simulink model "gm_final_heart_sym3_3_Level_fixed"  (R2021a)
settings: Solver=FixedStepDiscrete  StartTime=0.0  StopTime=8  RelTol=1e-3
libraries: hdlmdlgenlib x58
(part 2 of 3)

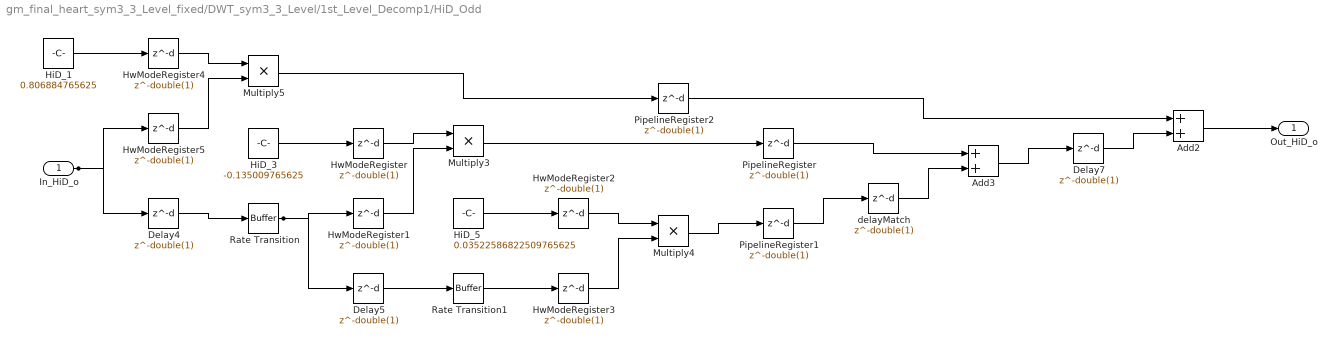
== system gm_final_heart_sym3_3_Level_fixed/DWT_sym3_3_Level/1st_Level_Decomp1/HiD_Odd ==
  In_HiD_o : Inport  OutDataTypeStr=fixdt(1, 16, 23)  PortDimensions=1  SampleTime=2.26757369614512e-05
  Add2 : Sum  AccumDataTypeStr=fixdt(1, 16, 23)  OutDataTypeStr=fixdt(1, 16, 24)  SampleTime=2.26757369614512e-05
  Add3 : Sum  AccumDataTypeStr=fixdt(1, 16, 26)  OutDataTypeStr=fixdt(1, 16, 26)  SampleTime=2.26757369614512e-05
  Delay4 : Delay  DelayLength=double(1)  InitialCondition=0  SampleTime=2.26757369614512e-05
  Delay5 : Delay  DelayLength=double(1)  InitialCondition=0  SampleTime=2.26757369614512e-05
  Delay7 : Delay  DelayLength=double(1)  InitialCondition=0  SampleTime=2.26757369614512e-05
  HiD_1 : Constant  Value=0.806884765625  OutDataTypeStr=fixdt(0, 16, 16)  SampleTime=2.26757369614512e-05
  HiD_3 : Constant  Value=-0.135009765625  OutDataTypeStr=fixdt(1, 16, 17)  SampleTime=2.26757369614512e-05
  HiD_5 : Constant  Value=0.03522586822509765625  OutDataTypeStr=fixdt(0, 16, 20)  SampleTime=2.26757369614512e-05
  HwModeRegister{,1..5} (6 alike) : Delay  DelayLength=double(1)  InitialCondition=0  SampleTime=2.26757369614512e-05
  Multiply3 : Product  Inputs=**  OutDataTypeStr=fixdt(1, 16, 15)  SampleTime=2.26757369614512e-05
  Multiply4 : Product  Inputs=**  OutDataTypeStr=fixdt(0, 16, 29)  SampleTime=2.26757369614512e-05
  Multiply5 : Product  Inputs=**  OutDataTypeStr=fixdt(0, 16, 24)  SampleTime=2.26757369614512e-05
  PipelineRegister : Delay  DelayLength=double(1)  InitialCondition=0  SampleTime=2.26757369614512e-05
  PipelineRegister1 : Delay  DelayLength=double(1)  InitialCondition=0  SampleTime=2.26757369614512e-05
  PipelineRegister2 : Delay  DelayLength=double(1)  InitialCondition=0  SampleTime=2.26757369614512e-05
  Rate Transition : hdlmdlgenlib/Buffer
      settings: SourceProductBaseCode=SL
  Rate Transition1 : hdlmdlgenlib/Buffer
      settings: SourceProductBaseCode=SL
  delayMatch : Delay  DelayLength=double(1)  InitialCondition=0  SampleTime=2.26757369614512e-05
  Out_HiD_o : Outport  OutDataTypeStr=fixdt(1,16,24)  SampleTime=2.26757369614512e-05  VectorParamsAs1DForOutWhenUnconnected=off
  wires:
  Add2/1 -> Out_HiD_o/1
  Add3/1 -> Delay7/1
  Delay4/1 -> Rate Transition/1
  Delay5/1 -> Rate Transition1/1
  Delay7/1 -> Add2/2
  HiD_1/1 -> HwModeRegister4/1
  HiD_3/1 -> HwModeRegister/1
  HiD_5/1 -> HwModeRegister2/1
  PipelineRegister/1 -> Add3/1
  delayMatch/1 -> Add3/2
  PipelineRegister2/1 -> Add2/1
  Rate Transition/1 -> Delay5/1, HwModeRegister1/1
  Rate Transition1/1 -> HwModeRegister3/1
  In_HiD_o/1 -> Delay4/1, HwModeRegister5/1
  PipelineRegister1/1 -> delayMatch/1
  Multiply3/1 -> PipelineRegister/1
  HwModeRegister/1 -> Multiply3/1
  HwModeRegister1/1 -> Multiply3/2
  Multiply4/1 -> PipelineRegister1/1
  HwModeRegister2/1 -> Multiply4/1
  HwModeRegister3/1 -> Multiply4/2
  Multiply5/1 -> PipelineRegister2/1
  HwModeRegister4/1 -> Multiply5/1
  HwModeRegister5/1 -> Multiply5/2

== system gm_final_heart_sym3_3_Level_fixed/DWT_sym3_3_Level/1st_Level_Decomp1/LoD_Even ==
  In_LoD_e : Inport  OutDataTypeStr=fixdt(1, 16, 23)  PortDimensions=1  SampleTime=2.26757369614512e-05
  Add2 : Sum  AccumDataTypeStr=fixdt(1, 16, 24)  OutDataTypeStr=fixdt(1, 16, 24)  SampleTime=2.26757369614512e-05
  Add3 : Sum  AccumDataTypeStr=fixdt(1, 16, 23)  OutDataTypeStr=fixdt(1, 16, 24)  SampleTime=2.26757369614512e-05
  Delay4 : Delay  DelayLength=double(1)  InitialCondition=0  SampleTime=2.26757369614512e-05
  Delay5 : Delay  DelayLength=double(1)  InitialCondition=0  SampleTime=2.26757369614512e-05
  Delay7 : Delay  DelayLength=double(1)  InitialCondition=0  SampleTime=2.26757369614512e-05
  HwModeRegister{,1..5} (6 alike) : Delay  DelayLength=double(1)  InitialCondition=0  SampleTime=2.26757369614512e-05
  LoD_1 : Constant  Value=0.03522586822509765625  OutDataTypeStr=fixdt(0, 16, 20)  SampleTime=2.26757369614512e-05
  LoD_3 : Constant  Value=-0.135009765625  OutDataTypeStr=fixdt(1, 16, 17)  SampleTime=2.26757369614512e-05
  LoD_5 : Constant  Value=0.806884765625  OutDataTypeStr=fixdt(0, 16, 16)  SampleTime=2.26757369614512e-05
  Multiply3 : Product  Inputs=**  OutDataTypeStr=fixdt(1, 16, 15)  SampleTime=2.26757369614512e-05
  Multiply4 : Product  Inputs=**  OutDataTypeStr=fixdt(0, 16, 24)  SampleTime=2.26757369614512e-05
  Multiply5 : Product  Inputs=**  OutDataTypeStr=fixdt(0, 16, 29)  SampleTime=2.26757369614512e-05
  PipelineRegister : Delay  DelayLength=double(1)  InitialCondition=0  SampleTime=2.26757369614512e-05
  PipelineRegister1 : Delay  DelayLength=double(1)  InitialCondition=0  SampleTime=2.26757369614512e-05
  PipelineRegister2 : Delay  DelayLength=double(1)  InitialCondition=0  SampleTime=2.26757369614512e-05
  Rate Transition : hdlmdlgenlib/Buffer
      settings: SourceProductBaseCode=SL
  Rate Transition1 : hdlmdlgenlib/Buffer
      settings: SourceProductBaseCode=SL
  delayMatch : Delay  DelayLength=double(1)  InitialCondition=0  SampleTime=2.26757369614512e-05
  Out_LoD_e : Outport  OutDataTypeStr=fixdt(1,16,24)  SampleTime=2.26757369614512e-05  VectorParamsAs1DForOutWhenUnconnected=off
  wires:
  Add2/1 -> Out_LoD_e/1
  Add3/1 -> Delay7/1
  Delay4/1 -> Rate Transition/1
  Delay5/1 -> Rate Transition1/1
  Delay7/1 -> Add2/2
  LoD_1/1 -> HwModeRegister4/1
  LoD_3/1 -> HwModeRegister/1
  LoD_5/1 -> HwModeRegister2/1
  PipelineRegister/1 -> Add3/1
  delayMatch/1 -> Add3/2
  PipelineRegister2/1 -> Add2/1
  Rate Transition/1 -> Delay5/1, HwModeRegister1/1
  Rate Transition1/1 -> HwModeRegister3/1
  In_LoD_e/1 -> Delay4/1, HwModeRegister5/1
  PipelineRegister1/1 -> delayMatch/1
  Multiply3/1 -> PipelineRegister/1
  HwModeRegister/1 -> Multiply3/1
  HwModeRegister1/1 -> Multiply3/2
  Multiply4/1 -> PipelineRegister1/1
  HwModeRegister2/1 -> Multiply4/1
  HwModeRegister3/1 -> Multiply4/2
  Multiply5/1 -> PipelineRegister2/1
  HwModeRegister4/1 -> Multiply5/1
  HwModeRegister5/1 -> Multiply5/2

== system gm_final_heart_sym3_3_Level_fixed/DWT_sym3_3_Level/1st_Level_Decomp1/LoD_Odd ==
  In_LoD_o : Inport  OutDataTypeStr=fixdt(1, 16, 23)  PortDimensions=1  SampleTime=2.26757369614512e-05
  Add2 : Sum  AccumDataTypeStr=fixdt(1, 16, 23)  OutDataTypeStr=fixdt(1, 16, 24)  SampleTime=2.26757369614512e-05
  Add3 : Sum  AccumDataTypeStr=fixdt(0, 16, 24)  OutDataTypeStr=fixdt(0, 16, 24)  SampleTime=2.26757369614512e-05
  Delay4 : Delay  DelayLength=double(1)  InitialCondition=0  SampleTime=2.26757369614512e-05
  Delay5 : Delay  DelayLength=double(1)  InitialCondition=0  SampleTime=2.26757369614512e-05
  Delay7 : Delay  DelayLength=double(1)  InitialCondition=0  SampleTime=2.26757369614512e-05
  HwModeRegister{,1..5} (6 alike) : Delay  DelayLength=double(1)  InitialCondition=0  SampleTime=2.26757369614512e-05
  LoD_1 : Constant  Value=-0.08544158935546875  OutDataTypeStr=fixdt(1, 16, 18)  SampleTime=2.26757369614512e-05
  LoD_3 : Constant  Value=0.45987701416015625  OutDataTypeStr=fixdt(0, 16, 17)  SampleTime=2.26757369614512e-05
  LoD_5 : Constant  Value=0.332672119140625  OutDataTypeStr=fixdt(0, 16, 17)  SampleTime=2.26757369614512e-05
  Multiply3 : Product  Inputs=**  OutDataTypeStr=fixdt(0, 16, 25)  SampleTime=2.26757369614512e-05
  Multiply4 : Product  Inputs=**  OutDataTypeStr=fixdt(0, 16, 26)  SampleTime=2.26757369614512e-05
  Multiply5 : Product  Inputs=**  OutDataTypeStr=fixdt(1, 16, 15)  SampleTime=2.26757369614512e-05
  PipelineRegister : Delay  DelayLength=double(1)  InitialCondition=0  SampleTime=2.26757369614512e-05
  PipelineRegister1 : Delay  DelayLength=double(1)  InitialCondition=0  SampleTime=2.26757369614512e-05
  PipelineRegister2 : Delay  DelayLength=double(1)  InitialCondition=0  SampleTime=2.26757369614512e-05
  Rate Transition : hdlmdlgenlib/Buffer
      settings: SourceProductBaseCode=SL
  Rate Transition1 : hdlmdlgenlib/Buffer
      settings: SourceProductBaseCode=SL
  delayMatch : Delay  DelayLength=double(1)  InitialCondition=0  SampleTime=2.26757369614512e-05
  Out_LoD_o : Outport  OutDataTypeStr=fixdt(1,16,24)  SampleTime=2.26757369614512e-05  VectorParamsAs1DForOutWhenUnconnected=off
  wires:
  Add2/1 -> Out_LoD_o/1
  Add3/1 -> Delay7/1
  Delay4/1 -> Rate Transition/1
  Delay5/1 -> Rate Transition1/1
  Delay7/1 -> Add2/2
  LoD_1/1 -> HwModeRegister4/1
  LoD_3/1 -> HwModeRegister/1
  LoD_5/1 -> HwModeRegister2/1
  PipelineRegister/1 -> Add3/1
  delayMatch/1 -> Add3/2
  PipelineRegister2/1 -> Add2/1
  Rate Transition/1 -> Delay5/1, HwModeRegister1/1
  Rate Transition1/1 -> HwModeRegister3/1
  In_LoD_o/1 -> Delay4/1, HwModeRegister5/1
  PipelineRegister1/1 -> delayMatch/1
  Multiply3/1 -> PipelineRegister/1
  HwModeRegister/1 -> Multiply3/1
  HwModeRegister1/1 -> Multiply3/2
  Multiply4/1 -> PipelineRegister1/1
  HwModeRegister2/1 -> Multiply4/1
  HwModeRegister3/1 -> Multiply4/2
  Multiply5/1 -> PipelineRegister2/1
  HwModeRegister4/1 -> Multiply5/1
  HwModeRegister5/1 -> Multiply5/2

== system gm_final_heart_sym3_3_Level_fixed/DWT_sym3_3_Level/1st_Level_Decomp2/HiD_Even ==
  In_HiD_e : Inport  OutDataTypeStr=fixdt(1, 16, 24)  PortDimensions=1  SampleTime=2.26757369614512e-05
  Add : Sum  AccumDataTypeStr=fixdt(1, 16, 24)  OutDataTypeStr=fixdt(1, 16, 24)  SampleTime=2.26757369614512e-05
  Add1 : Sum  AccumDataTypeStr=fixdt(1, 16, 25)  OutDataTypeStr=fixdt(1, 16, 25)  SampleTime=2.26757369614512e-05
  Delay : Delay  DelayLength=double(1)  InitialCondition=0  SampleTime=2.26757369614512e-05
  Delay1 : Delay  DelayLength=double(1)  InitialCondition=0  SampleTime=2.26757369614512e-05
  Delay3 : Delay  DelayLength=double(1)  InitialCondition=0  SampleTime=2.26757369614512e-05
  HiD_0 : Constant  Value=-0.332672119140625  OutDataTypeStr=fixdt(1, 16, 16)  SampleTime=2.26757369614512e-05
  HiD_2 : Constant  Value=-0.4598846435546875  OutDataTypeStr=fixdt(1, 16, 16)  SampleTime=2.26757369614512e-05
  HiD_4 : Constant  Value=0.08544158935546875  OutDataTypeStr=fixdt(0, 16, 19)  SampleTime=2.26757369614512e-05
  HwModeRegister{,1..5} (6 alike) : Delay  DelayLength=double(1)  InitialCondition=0  SampleTime=2.26757369614512e-05
  Multiply1 : Product  Inputs=**  OutDataTypeStr=fixdt(1, 16, 15)  SampleTime=2.26757369614512e-05
  Multiply2 : Product  Inputs=**  OutDataTypeStr=fixdt(0, 16, 28)  SampleTime=2.26757369614512e-05
  Multiply3 : Product  Inputs=**  OutDataTypeStr=fixdt(1, 16, 15)  SampleTime=2.26757369614512e-05
  PipelineRegister : Delay  DelayLength=double(1)  InitialCondition=0  SampleTime=2.26757369614512e-05
  PipelineRegister1 : Delay  DelayLength=double(1)  InitialCondition=0  SampleTime=2.26757369614512e-05
  PipelineRegister2 : Delay  DelayLength=double(1)  InitialCondition=0  SampleTime=2.26757369614512e-05
  Rate Transition : hdlmdlgenlib/Buffer
      settings: SourceProductBaseCode=SL
  Rate Transition1 : hdlmdlgenlib/Buffer
      settings: SourceProductBaseCode=SL
  delayMatch : Delay  DelayLength=double(1)  InitialCondition=0  SampleTime=2.26757369614512e-05
  Out_HiD_e : Outport  OutDataTypeStr=fixdt(1,16,24)  SampleTime=2.26757369614512e-05  VectorParamsAs1DForOutWhenUnconnected=off
  wires:
  Add/1 -> Out_HiD_e/1
  Add1/1 -> Delay3/1
  Delay/1 -> Rate Transition/1
  Delay1/1 -> Rate Transition1/1
  Delay3/1 -> Add/2
  HiD_0/1 -> HwModeRegister4/1
  HiD_2/1 -> HwModeRegister/1
  HiD_4/1 -> HwModeRegister2/1
  PipelineRegister/1 -> Add1/1
  delayMatch/1 -> Add1/2
  PipelineRegister2/1 -> Add/1
  Rate Transition/1 -> Delay1/1, HwModeRegister1/1
  Rate Transition1/1 -> HwModeRegister3/1
  In_HiD_e/1 -> Delay/1, HwModeRegister5/1
  PipelineRegister1/1 -> delayMatch/1
  Multiply1/1 -> PipelineRegister/1
  HwModeRegister/1 -> Multiply1/1
  HwModeRegister1/1 -> Multiply1/2
  Multiply2/1 -> PipelineRegister1/1
  HwModeRegister2/1 -> Multiply2/1
  HwModeRegister3/1 -> Multiply2/2
  Multiply3/1 -> PipelineRegister2/1
  HwModeRegister4/1 -> Multiply3/1
  HwModeRegister5/1 -> Multiply3/2

== system gm_final_heart_sym3_3_Level_fixed/DWT_sym3_3_Level/1st_Level_Decomp2/HiD_Odd ==
  In_HiD_o : Inport  OutDataTypeStr=fixdt(1, 16, 24)  PortDimensions=1  SampleTime=2.26757369614512e-05
  Add2 : Sum  AccumDataTypeStr=fixdt(1, 16, 24)  OutDataTypeStr=fixdt(1, 16, 24)  SampleTime=2.26757369614512e-05
  Add3 : Sum  AccumDataTypeStr=fixdt(1, 16, 26)  OutDataTypeStr=fixdt(1, 16, 27)  SampleTime=2.26757369614512e-05
  Delay4 : Delay  DelayLength=double(1)  InitialCondition=0  SampleTime=2.26757369614512e-05
  Delay5 : Delay  DelayLength=double(1)  InitialCondition=0  SampleTime=2.26757369614512e-05
  Delay7 : Delay  DelayLength=double(1)  InitialCondition=0  SampleTime=2.26757369614512e-05
  HiD_1 : Constant  Value=0.806884765625  OutDataTypeStr=fixdt(0, 16, 16)  SampleTime=2.26757369614512e-05
  HiD_3 : Constant  Value=-0.135009765625  OutDataTypeStr=fixdt(1, 16, 17)  SampleTime=2.26757369614512e-05
  HiD_5 : Constant  Value=0.03522586822509765625  OutDataTypeStr=fixdt(0, 16, 20)  SampleTime=2.26757369614512e-05
  HwModeRegister{,1..5} (6 alike) : Delay  DelayLength=double(1)  InitialCondition=0  SampleTime=2.26757369614512e-05
  Multiply3 : Product  Inputs=**  OutDataTypeStr=fixdt(1, 16, 15)  SampleTime=2.26757369614512e-05
  Multiply4 : Product  Inputs=**  OutDataTypeStr=fixdt(0, 16, 29)  SampleTime=2.26757369614512e-05
  Multiply5 : Product  Inputs=**  OutDataTypeStr=fixdt(0, 16, 25)  SampleTime=2.26757369614512e-05
  PipelineRegister : Delay  DelayLength=double(1)  InitialCondition=0  SampleTime=2.26757369614512e-05
  PipelineRegister1 : Delay  DelayLength=double(1)  InitialCondition=0  SampleTime=2.26757369614512e-05
  PipelineRegister2 : Delay  DelayLength=double(1)  InitialCondition=0  SampleTime=2.26757369614512e-05
  Rate Transition : hdlmdlgenlib/Buffer
      settings: SourceProductBaseCode=SL
  Rate Transition1 : hdlmdlgenlib/Buffer
      settings: SourceProductBaseCode=SL
  delayMatch : Delay  DelayLength=double(1)  InitialCondition=0  SampleTime=2.26757369614512e-05
  Out_HiD_o : Outport  OutDataTypeStr=fixdt(1,16,24)  SampleTime=2.26757369614512e-05  VectorParamsAs1DForOutWhenUnconnected=off
  wires:
  Add2/1 -> Out_HiD_o/1
  Add3/1 -> Delay7/1
  Delay4/1 -> Rate Transition/1
  Delay5/1 -> Rate Transition1/1
  Delay7/1 -> Add2/2
  HiD_1/1 -> HwModeRegister4/1
  HiD_3/1 -> HwModeRegister/1
  HiD_5/1 -> HwModeRegister2/1
  PipelineRegister/1 -> Add3/1
  delayMatch/1 -> Add3/2
  PipelineRegister2/1 -> Add2/1
  Rate Transition/1 -> Delay5/1, HwModeRegister1/1
  Rate Transition1/1 -> HwModeRegister3/1
  In_HiD_o/1 -> Delay4/1, HwModeRegister5/1
  PipelineRegister1/1 -> delayMatch/1
  Multiply3/1 -> PipelineRegister/1
  HwModeRegister/1 -> Multiply3/1
  HwModeRegister1/1 -> Multiply3/2
  Multiply4/1 -> PipelineRegister1/1
  HwModeRegister2/1 -> Multiply4/1
  HwModeRegister3/1 -> Multiply4/2
  Multiply5/1 -> PipelineRegister2/1
  HwModeRegister4/1 -> Multiply5/1
  HwModeRegister5/1 -> Multiply5/2

== system gm_final_heart_sym3_3_Level_fixed/DWT_sym3_3_Level/1st_Level_Decomp2/LoD_Even ==
  In_LoD_e : Inport  OutDataTypeStr=fixdt(1, 16, 24)  PortDimensions=1  SampleTime=2.26757369614512e-05
  Add2 : Sum  AccumDataTypeStr=fixdt(1, 16, 24)  OutDataTypeStr=fixdt(1, 16, 24)  SampleTime=2.26757369614512e-05
  Add3 : Sum  AccumDataTypeStr=fixdt(1, 16, 24)  OutDataTypeStr=fixdt(1, 16, 24)  SampleTime=2.26757369614512e-05
  Delay4 : Delay  DelayLength=double(1)  InitialCondition=0  SampleTime=2.26757369614512e-05
  Delay5 : Delay  DelayLength=double(1)  InitialCondition=0  SampleTime=2.26757369614512e-05
  Delay7 : Delay  DelayLength=double(1)  InitialCondition=0  SampleTime=2.26757369614512e-05
  HwModeRegister{,1..5} (6 alike) : Delay  DelayLength=double(1)  InitialCondition=0  SampleTime=2.26757369614512e-05
  LoD_1 : Constant  Value=0.03522586822509765625  OutDataTypeStr=fixdt(0, 16, 20)  SampleTime=2.26757369614512e-05
  LoD_3 : Constant  Value=-0.135009765625  OutDataTypeStr=fixdt(1, 16, 17)  SampleTime=2.26757369614512e-05
  LoD_5 : Constant  Value=0.806884765625  OutDataTypeStr=fixdt(0, 16, 16)  SampleTime=2.26757369614512e-05
  Multiply3 : Product  Inputs=**  OutDataTypeStr=fixdt(1, 16, 15)  SampleTime=2.26757369614512e-05
  Multiply4 : Product  Inputs=**  OutDataTypeStr=fixdt(0, 16, 25)  SampleTime=2.26757369614512e-05
  Multiply5 : Product  Inputs=**  OutDataTypeStr=fixdt(0, 16, 29)  SampleTime=2.26757369614512e-05
  PipelineRegister : Delay  DelayLength=double(1)  InitialCondition=0  SampleTime=2.26757369614512e-05
  PipelineRegister1 : Delay  DelayLength=double(1)  InitialCondition=0  SampleTime=2.26757369614512e-05
  PipelineRegister2 : Delay  DelayLength=double(1)  InitialCondition=0  SampleTime=2.26757369614512e-05
  Rate Transition : hdlmdlgenlib/Buffer
      settings: SourceProductBaseCode=SL
  Rate Transition1 : hdlmdlgenlib/Buffer
      settings: SourceProductBaseCode=SL
  delayMatch : Delay  DelayLength=double(1)  InitialCondition=0  SampleTime=2.26757369614512e-05
  Out_LoD_e : Outport  OutDataTypeStr=fixdt(1,16,24)  SampleTime=2.26757369614512e-05  VectorParamsAs1DForOutWhenUnconnected=off
  wires:
  Add2/1 -> Out_LoD_e/1
  Add3/1 -> Delay7/1
  Delay4/1 -> Rate Transition/1
  Delay5/1 -> Rate Transition1/1
  Delay7/1 -> Add2/2
  LoD_1/1 -> HwModeRegister4/1
  LoD_3/1 -> HwModeRegister/1
  LoD_5/1 -> HwModeRegister2/1
  PipelineRegister/1 -> Add3/1
  delayMatch/1 -> Add3/2
  PipelineRegister2/1 -> Add2/1
  Rate Transition/1 -> Delay5/1, HwModeRegister1/1
  Rate Transition1/1 -> HwModeRegister3/1
  In_LoD_e/1 -> Delay4/1, HwModeRegister5/1
  PipelineRegister1/1 -> delayMatch/1
  Multiply3/1 -> PipelineRegister/1
  HwModeRegister/1 -> Multiply3/1
  HwModeRegister1/1 -> Multiply3/2
  Multiply4/1 -> PipelineRegister1/1
  HwModeRegister2/1 -> Multiply4/1
  HwModeRegister3/1 -> Multiply4/2
  Multiply5/1 -> PipelineRegister2/1
  HwModeRegister4/1 -> Multiply5/1
  HwModeRegister5/1 -> Multiply5/2

== system gm_final_heart_sym3_3_Level_fixed/DWT_sym3_3_Level/1st_Level_Decomp2/LoD_Odd ==
  In_LoD_o : Inport  OutDataTypeStr=fixdt(1, 16, 24)  PortDimensions=1  SampleTime=2.26757369614512e-05
  Add2 : Sum  AccumDataTypeStr=fixdt(1, 16, 24)  OutDataTypeStr=fixdt(1, 16, 24)  SampleTime=2.26757369614512e-05
  Add3 : Sum  AccumDataTypeStr=fixdt(0, 16, 25)  OutDataTypeStr=fixdt(0, 16, 25)  SampleTime=2.26757369614512e-05
  Delay4 : Delay  DelayLength=double(1)  InitialCondition=0  SampleTime=2.26757369614512e-05
  Delay5 : Delay  DelayLength=double(1)  InitialCondition=0  SampleTime=2.26757369614512e-05
  Delay7 : Delay  DelayLength=double(1)  InitialCondition=0  SampleTime=2.26757369614512e-05
  HwModeRegister{,1..5} (6 alike) : Delay  DelayLength=double(1)  InitialCondition=0  SampleTime=2.26757369614512e-05
  LoD_1 : Constant  Value=-0.08544158935546875  OutDataTypeStr=fixdt(1, 16, 18)  SampleTime=2.26757369614512e-05
  LoD_3 : Constant  Value=0.45987701416015625  OutDataTypeStr=fixdt(0, 16, 17)  SampleTime=2.26757369614512e-05
  LoD_5 : Constant  Value=0.332672119140625  OutDataTypeStr=fixdt(0, 16, 17)  SampleTime=2.26757369614512e-05
  Multiply3 : Product  Inputs=**  OutDataTypeStr=fixdt(0, 16, 26)  SampleTime=2.26757369614512e-05
  Multiply4 : Product  Inputs=**  OutDataTypeStr=fixdt(0, 16, 26)  SampleTime=2.26757369614512e-05
  Multiply5 : Product  Inputs=**  OutDataTypeStr=fixdt(1, 16, 15)  SampleTime=2.26757369614512e-05
  PipelineRegister : Delay  DelayLength=double(1)  InitialCondition=0  SampleTime=2.26757369614512e-05
  PipelineRegister1 : Delay  DelayLength=double(1)  InitialCondition=0  SampleTime=2.26757369614512e-05
  PipelineRegister2 : Delay  DelayLength=double(1)  InitialCondition=0  SampleTime=2.26757369614512e-05
  Rate Transition : hdlmdlgenlib/Buffer
      settings: SourceProductBaseCode=SL
  Rate Transition1 : hdlmdlgenlib/Buffer
      settings: SourceProductBaseCode=SL
  delayMatch : Delay  DelayLength=double(1)  InitialCondition=0  SampleTime=2.26757369614512e-05
  Out_LoD_o : Outport  OutDataTypeStr=fixdt(1,16,24)  SampleTime=2.26757369614512e-05  VectorParamsAs1DForOutWhenUnconnected=off
  wires:
  Add2/1 -> Out_LoD_o/1
  Add3/1 -> Delay7/1
  Delay4/1 -> Rate Transition/1
  Delay5/1 -> Rate Transition1/1
  Delay7/1 -> Add2/2
  LoD_1/1 -> HwModeRegister4/1
  LoD_3/1 -> HwModeRegister/1
  LoD_5/1 -> HwModeRegister2/1
  PipelineRegister/1 -> Add3/1
  delayMatch/1 -> Add3/2
  PipelineRegister2/1 -> Add2/1
  Rate Transition/1 -> Delay5/1, HwModeRegister1/1
  Rate Transition1/1 -> HwModeRegister3/1
  In_LoD_o/1 -> Delay4/1, HwModeRegister5/1
  PipelineRegister1/1 -> delayMatch/1
  Multiply3/1 -> PipelineRegister/1
  HwModeRegister/1 -> Multiply3/1
  HwModeRegister1/1 -> Multiply3/2
  Multiply4/1 -> PipelineRegister1/1
  HwModeRegister2/1 -> Multiply4/1
  HwModeRegister3/1 -> Multiply4/2
  Multiply5/1 -> PipelineRegister2/1
  HwModeRegister4/1 -> Multiply5/1
  HwModeRegister5/1 -> Multiply5/2

== system gm_final_heart_sym3_3_Level_fixed/DWT_sym3_3_Level/1st_Level_Recon/HiR_Even ==
  In_HiR_e : Inport  OutDataTypeStr=fixdt(1, 16, 28)  PortDimensions=1  SampleTime=2.26757369614512e-05
  Add : Sum  AccumDataTypeStr=fixdt(1, 16, 28)  OutDataTypeStr=fixdt(1, 16, 28)  SampleTime=2.26757369614512e-05
  Add1 : Sum  AccumDataTypeStr=fixdt(1, 16, 28)  OutDataTypeStr=fixdt(1, 16, 28)  SampleTime=2.26757369614512e-05
  Delay : Delay  DelayLength=double(1)  InitialCondition=0  SampleTime=2.26757369614512e-05
  Delay1 : Delay  DelayLength=double(1)  InitialCondition=0  SampleTime=2.26757369614512e-05
  Delay3 : Delay  DelayLength=double(1)  InitialCondition=0  SampleTime=2.26757369614512e-05
  HiR_0 : Constant  Value=0.03522586822509765625  OutDataTypeStr=fixdt(0, 16, 20)  SampleTime=2.26757369614512e-05
  HiR_2 : Constant  Value=-0.135009765625  OutDataTypeStr=fixdt(1, 16, 17)  SampleTime=2.26757369614512e-05
  HiR_4 : Constant  Value=0.806884765625  OutDataTypeStr=fixdt(0, 16, 16)  SampleTime=2.26757369614512e-05
  HwModeRegister{,1..5} (6 alike) : Delay  DelayLength=double(1)  InitialCondition=0  SampleTime=2.26757369614512e-05
  Multiply : Product  Inputs=**  OutDataTypeStr=fixdt(1, 16, 33)  SampleTime=2.26757369614512e-05
  Multiply1 : Product  Inputs=**  OutDataTypeStr=fixdt(1, 16, 31)  SampleTime=2.26757369614512e-05
  Multiply2 : Product  Inputs=**  OutDataTypeStr=fixdt(1, 16, 28)  SampleTime=2.26757369614512e-05
  PipelineRegister : Delay  DelayLength=double(1)  InitialCondition=0  SampleTime=2.26757369614512e-05
  PipelineRegister1 : Delay  DelayLength=double(1)  InitialCondition=0  SampleTime=2.26757369614512e-05
  PipelineRegister2 : Delay  DelayLength=double(1)  InitialCondition=0  SampleTime=2.26757369614512e-05
  Rate Transition : hdlmdlgenlib/Buffer
      settings: SourceProductBaseCode=SL
  Rate Transition1 : hdlmdlgenlib/Buffer
      settings: SourceProductBaseCode=SL
  delayMatch : Delay  DelayLength=double(1)  InitialCondition=0  SampleTime=2.26757369614512e-05
  Out_HiR_e : Outport  OutDataTypeStr=fixdt(1,16,28)  SampleTime=2.26757369614512e-05  VectorParamsAs1DForOutWhenUnconnected=off
  wires:
  Add/1 -> Out_HiR_e/1
  Add1/1 -> Delay3/1
  Delay/1 -> Rate Transition/1
  Delay1/1 -> Rate Transition1/1
  Delay3/1 -> Add/2
  HiR_0/1 -> HwModeRegister/1
  HiR_2/1 -> HwModeRegister2/1
  HiR_4/1 -> HwModeRegister4/1
  PipelineRegister/1 -> Add/1
  PipelineRegister1/1 -> Add1/1
  delayMatch/1 -> Add1/2
  Rate Transition/1 -> Delay1/1, HwModeRegister3/1
  Rate Transition1/1 -> HwModeRegister5/1
  In_HiR_e/1 -> Delay/1, HwModeRegister1/1
  PipelineRegister2/1 -> delayMatch/1
  Multiply/1 -> PipelineRegister/1
  HwModeRegister/1 -> Multiply/1
  HwModeRegister1/1 -> Multiply/2
  Multiply1/1 -> PipelineRegister1/1
  HwModeRegister2/1 -> Multiply1/1
  HwModeRegister3/1 -> Multiply1/2
  Multiply2/1 -> PipelineRegister2/1
  HwModeRegister4/1 -> Multiply2/1
  HwModeRegister5/1 -> Multiply2/2

== system gm_final_heart_sym3_3_Level_fixed/DWT_sym3_3_Level/1st_Level_Recon/HiR_Odd ==
  In_HiR_o : Inport  OutDataTypeStr=fixdt(1, 16, 28)  PortDimensions=1  SampleTime=2.26757369614512e-05
  Add : Sum  AccumDataTypeStr=fixdt(1, 16, 29)  OutDataTypeStr=fixdt(1, 16, 29)  SampleTime=2.26757369614512e-05
  Add1 : Sum  AccumDataTypeStr=fixdt(1, 16, 29)  OutDataTypeStr=fixdt(1, 16, 29)  SampleTime=2.26757369614512e-05
  Delay : Delay  DelayLength=double(1)  InitialCondition=0  SampleTime=2.26757369614512e-05
  Delay1 : Delay  DelayLength=double(1)  InitialCondition=0  SampleTime=2.26757369614512e-05
  Delay3 : Delay  DelayLength=double(1)  InitialCondition=0  SampleTime=2.26757369614512e-05
  HiR_1 : Constant  Value=0.08544158935546875  OutDataTypeStr=fixdt(0, 16, 19)  SampleTime=2.26757369614512e-05
  HiR_3 : Constant  Value=-0.4598846435546875  OutDataTypeStr=fixdt(1, 16, 16)  SampleTime=2.26757369614512e-05
  HiR_5 : Constant  Value=-0.332672119140625  OutDataTypeStr=fixdt(1, 16, 16)  SampleTime=2.26757369614512e-05
  HwModeRegister{,1..5} (6 alike) : Delay  DelayLength=double(1)  InitialCondition=0  SampleTime=2.26757369614512e-05
  Multiply : Product  Inputs=**  OutDataTypeStr=fixdt(1, 16, 31)  SampleTime=2.26757369614512e-05
  Multiply1 : Product  Inputs=**  OutDataTypeStr=fixdt(1, 16, 29)  SampleTime=2.26757369614512e-05
  Multiply2 : Product  Inputs=**  OutDataTypeStr=fixdt(1, 16, 30)  SampleTime=2.26757369614512e-05
  PipelineRegister : Delay  DelayLength=double(1)  InitialCondition=0  SampleTime=2.26757369614512e-05
  PipelineRegister1 : Delay  DelayLength=double(1)  InitialCondition=0  SampleTime=2.26757369614512e-05
  PipelineRegister2 : Delay  DelayLength=double(1)  InitialCondition=0  SampleTime=2.26757369614512e-05
  Rate Transition : hdlmdlgenlib/Buffer
      settings: SourceProductBaseCode=SL
  Rate Transition1 : hdlmdlgenlib/Buffer
      settings: SourceProductBaseCode=SL
  delayMatch : Delay  DelayLength=double(1)  InitialCondition=0  SampleTime=2.26757369614512e-05
  Out_HiR_o : Outport  OutDataTypeStr=fixdt(1,16,29)  SampleTime=2.26757369614512e-05  VectorParamsAs1DForOutWhenUnconnected=off
  wires:
  Add/1 -> Out_HiR_o/1
  Add1/1 -> Delay3/1
  Delay/1 -> Rate Transition/1
  Delay1/1 -> Rate Transition1/1
  Delay3/1 -> Add/2
  HiR_1/1 -> HwModeRegister/1
  HiR_3/1 -> HwModeRegister2/1
  HiR_5/1 -> HwModeRegister4/1
  PipelineRegister/1 -> Add/1
  PipelineRegister1/1 -> Add1/1
  delayMatch/1 -> Add1/2
  Rate Transition/1 -> Delay1/1, HwModeRegister3/1
  Rate Transition1/1 -> HwModeRegister5/1
  In_HiR_o/1 -> Delay/1, HwModeRegister1/1
  PipelineRegister2/1 -> delayMatch/1
  Multiply/1 -> PipelineRegister/1
  HwModeRegister/1 -> Multiply/1
  HwModeRegister1/1 -> Multiply/2
  Multiply1/1 -> PipelineRegister1/1
  HwModeRegister2/1 -> Multiply1/1
  HwModeRegister3/1 -> Multiply1/2
  Multiply2/1 -> PipelineRegister2/1
  HwModeRegister4/1 -> Multiply2/1
  HwModeRegister5/1 -> Multiply2/2

== system gm_final_heart_sym3_3_Level_fixed/DWT_sym3_3_Level/1st_Level_Recon/LoR_Even ==
  In_LoR_e : Inport  OutDataTypeStr=fixdt(1, 16, 24)  PortDimensions=1  SampleTime=2.26757369614512e-05
  Add : Sum  AccumDataTypeStr=fixdt(1, 16, 24)  OutDataTypeStr=fixdt(1, 16, 24)  SampleTime=2.26757369614512e-05
  Add1 : Sum  AccumDataTypeStr=fixdt(1, 16, 25)  OutDataTypeStr=fixdt(1, 16, 25)  SampleTime=2.26757369614512e-05
  Delay : Delay  DelayLength=double(1)  InitialCondition=0  SampleTime=2.26757369614512e-05
  Delay1 : Delay  DelayLength=double(1)  InitialCondition=0  SampleTime=2.26757369614512e-05
  Delay3 : Delay  DelayLength=double(1)  InitialCondition=0  SampleTime=2.26757369614512e-05
  HwModeRegister{,1..5} (6 alike) : Delay  DelayLength=double(1)  InitialCondition=0  SampleTime=2.26757369614512e-05
  LoR_0 : Constant  Value=0.332672119140625  OutDataTypeStr=fixdt(0, 16, 17)  SampleTime=2.26757369614512e-05
  LoR_2 : Constant  Value=0.45987701416015625  OutDataTypeStr=fixdt(0, 16, 17)  SampleTime=2.26757369614512e-05
  LoR_4 : Constant  Value=-0.08544158935546875  OutDataTypeStr=fixdt(1, 16, 18)  SampleTime=2.26757369614512e-05
  Multiply : Product  Inputs=**  OutDataTypeStr=fixdt(1, 16, 26)  SampleTime=2.26757369614512e-05
  Multiply1 : Product  Inputs=**  OutDataTypeStr=fixdt(1, 16, 25)  SampleTime=2.26757369614512e-05
  Multiply2 : Product  Inputs=**  OutDataTypeStr=fixdt(1, 16, 27)  SampleTime=2.26757369614512e-05
  PipelineRegister : Delay  DelayLength=double(1)  InitialCondition=0  SampleTime=2.26757369614512e-05
  PipelineRegister1 : Delay  DelayLength=double(1)  InitialCondition=0  SampleTime=2.26757369614512e-05
  PipelineRegister2 : Delay  DelayLength=double(1)  InitialCondition=0  SampleTime=2.26757369614512e-05
  Rate Transition : hdlmdlgenlib/Buffer
      settings: SourceProductBaseCode=SL
  Rate Transition1 : hdlmdlgenlib/Buffer
      settings: SourceProductBaseCode=SL
  delayMatch : Delay  DelayLength=double(1)  InitialCondition=0  SampleTime=2.26757369614512e-05
  Out_LoR_e : Outport  OutDataTypeStr=fixdt(1,16,24)  SampleTime=2.26757369614512e-05  VectorParamsAs1DForOutWhenUnconnected=off
  wires:
  Add/1 -> Out_LoR_e/1
  Add1/1 -> Delay3/1
  Delay/1 -> Rate Transition/1
  Delay1/1 -> Rate Transition1/1
  Delay3/1 -> Add/2
  LoR_0/1 -> HwModeRegister/1
  LoR_2/1 -> HwModeRegister2/1
  LoR_4/1 -> HwModeRegister4/1
  PipelineRegister/1 -> Add/1
  PipelineRegister1/1 -> Add1/1
  delayMatch/1 -> Add1/2
  Rate Transition/1 -> Delay1/1, HwModeRegister3/1
  Rate Transition1/1 -> HwModeRegister5/1
  In_LoR_e/1 -> Delay/1, HwModeRegister1/1
  PipelineRegister2/1 -> delayMatch/1
  Multiply/1 -> PipelineRegister/1
  HwModeRegister/1 -> Multiply/1
  HwModeRegister1/1 -> Multiply/2
  Multiply1/1 -> PipelineRegister1/1
  HwModeRegister2/1 -> Multiply1/1
  HwModeRegister3/1 -> Multiply1/2
  Multiply2/1 -> PipelineRegister2/1
  HwModeRegister4/1 -> Multiply2/1
  HwModeRegister5/1 -> Multiply2/2

== system gm_final_heart_sym3_3_Level_fixed/DWT_sym3_3_Level/1st_Level_Recon/LoR_Odd ==
  In_LoR_o : Inport  OutDataTypeStr=fixdt(1, 16, 24)  PortDimensions=1  SampleTime=2.26757369614512e-05
  Add : Sum  AccumDataTypeStr=fixdt(1, 16, 24)  OutDataTypeStr=fixdt(1, 16, 24)  SampleTime=2.26757369614512e-05
  Add1 : Sum  AccumDataTypeStr=fixdt(1, 16, 27)  OutDataTypeStr=fixdt(1, 16, 27)  SampleTime=2.26757369614512e-05
  Delay : Delay  DelayLength=double(1)  InitialCondition=0  SampleTime=2.26757369614512e-05
  Delay1 : Delay  DelayLength=double(1)  InitialCondition=0  SampleTime=2.26757369614512e-05
  Delay3 : Delay  DelayLength=double(1)  InitialCondition=0  SampleTime=2.26757369614512e-05
  HwModeRegister{,1..5} (6 alike) : Delay  DelayLength=double(1)  InitialCondition=0  SampleTime=2.26757369614512e-05
  LoR_1 : Constant  Value=0.806884765625  OutDataTypeStr=fixdt(0, 16, 16)  SampleTime=2.26757369614512e-05
  LoR_3 : Constant  Value=-0.135009765625  OutDataTypeStr=fixdt(1, 16, 17)  SampleTime=2.26757369614512e-05
  LoR_5 : Constant  Value=0.03522586822509765625  OutDataTypeStr=fixdt(0, 16, 20)  SampleTime=2.26757369614512e-05
  Multiply : Product  Inputs=**  OutDataTypeStr=fixdt(1, 16, 24)  SampleTime=2.26757369614512e-05
  Multiply1 : Product  Inputs=**  OutDataTypeStr=fixdt(1, 16, 27)  SampleTime=2.26757369614512e-05
  Multiply2 : Product  Inputs=**  OutDataTypeStr=fixdt(1, 16, 29)  SampleTime=2.26757369614512e-05
  PipelineRegister : Delay  DelayLength=double(1)  InitialCondition=0  SampleTime=2.26757369614512e-05
  PipelineRegister1 : Delay  DelayLength=double(1)  InitialCondition=0  SampleTime=2.26757369614512e-05
  PipelineRegister2 : Delay  DelayLength=double(1)  InitialCondition=0  SampleTime=2.26757369614512e-05
  Rate Transition : hdlmdlgenlib/Buffer
      settings: SourceProductBaseCode=SL
  Rate Transition1 : hdlmdlgenlib/Buffer
      settings: SourceProductBaseCode=SL
  delayMatch : Delay  DelayLength=double(1)  InitialCondition=0  SampleTime=2.26757369614512e-05
  Out_LoR_o : Outport  OutDataTypeStr=fixdt(1,16,24)  SampleTime=2.26757369614512e-05  VectorParamsAs1DForOutWhenUnconnected=off
  wires:
  Add/1 -> Out_LoR_o/1
  Add1/1 -> Delay3/1
  Delay/1 -> Rate Transition/1
  Delay1/1 -> Rate Transition1/1
  Delay3/1 -> Add/2
  LoR_1/1 -> HwModeRegister/1
  LoR_3/1 -> HwModeRegister2/1
  LoR_5/1 -> HwModeRegister4/1
  PipelineRegister/1 -> Add/1
  PipelineRegister1/1 -> Add1/1
  delayMatch/1 -> Add1/2
  Rate Transition/1 -> Delay1/1, HwModeRegister3/1
  Rate Transition1/1 -> HwModeRegister5/1
  In_LoR_o/1 -> Delay/1, HwModeRegister1/1
  PipelineRegister2/1 -> delayMatch/1
  Multiply/1 -> PipelineRegister/1
  HwModeRegister/1 -> Multiply/1
  HwModeRegister1/1 -> Multiply/2
  Multiply1/1 -> PipelineRegister1/1
  HwModeRegister2/1 -> Multiply1/1
  HwModeRegister3/1 -> Multiply1/2
  Multiply2/1 -> PipelineRegister2/1
  HwModeRegister4/1 -> Multiply2/1
  HwModeRegister5/1 -> Multiply2/2

== system gm_final_heart_sym3_3_Level_fixed/DWT_sym3_3_Level/1st_Level_Recon1/HiR_Even ==
  In_HiR_e : Inport  OutDataTypeStr=fixdt(1, 16, 28)  PortDimensions=1  SampleTime=2.26757369614512e-05
  Add : Sum  AccumDataTypeStr=fixdt(1, 16, 28)  OutDataTypeStr=fixdt(1, 16, 28)  SampleTime=2.26757369614512e-05
  Add1 : Sum  AccumDataTypeStr=fixdt(1, 16, 28)  OutDataTypeStr=fixdt(1, 16, 28)  SampleTime=2.26757369614512e-05
  Delay : Delay  DelayLength=double(1)  InitialCondition=0  SampleTime=2.26757369614512e-05
  Delay1 : Delay  DelayLength=double(1)  InitialCondition=0  SampleTime=2.26757369614512e-05
  Delay3 : Delay  DelayLength=double(1)  InitialCondition=0  SampleTime=2.26757369614512e-05
  HiR_0 : Constant  Value=0.03522586822509765625  OutDataTypeStr=fixdt(0, 16, 20)  SampleTime=2.26757369614512e-05
  HiR_2 : Constant  Value=-0.135009765625  OutDataTypeStr=fixdt(1, 16, 17)  SampleTime=2.26757369614512e-05
  HiR_4 : Constant  Value=0.806884765625  OutDataTypeStr=fixdt(0, 16, 16)  SampleTime=2.26757369614512e-05
  HwModeRegister{,1..5} (6 alike) : Delay  DelayLength=double(1)  InitialCondition=0  SampleTime=2.26757369614512e-05
  Multiply : Product  Inputs=**  OutDataTypeStr=fixdt(1, 16, 33)  SampleTime=2.26757369614512e-05
  Multiply1 : Product  Inputs=**  OutDataTypeStr=fixdt(1, 16, 31)  SampleTime=2.26757369614512e-05
  Multiply2 : Product  Inputs=**  OutDataTypeStr=fixdt(1, 16, 28)  SampleTime=2.26757369614512e-05
  PipelineRegister : Delay  DelayLength=double(1)  InitialCondition=0  SampleTime=2.26757369614512e-05
  PipelineRegister1 : Delay  DelayLength=double(1)  InitialCondition=0  SampleTime=2.26757369614512e-05
  PipelineRegister2 : Delay  DelayLength=double(1)  InitialCondition=0  SampleTime=2.26757369614512e-05
  Rate Transition : hdlmdlgenlib/Buffer
      settings: SourceProductBaseCode=SL
  Rate Transition1 : hdlmdlgenlib/Buffer
      settings: SourceProductBaseCode=SL
  delayMatch : Delay  DelayLength=double(1)  InitialCondition=0  SampleTime=2.26757369614512e-05
  Out_HiR_e : Outport  OutDataTypeStr=fixdt(1,16,28)  SampleTime=2.26757369614512e-05  VectorParamsAs1DForOutWhenUnconnected=off
  wires:
  Add/1 -> Out_HiR_e/1
  Add1/1 -> Delay3/1
  Delay/1 -> Rate Transition/1
  Delay1/1 -> Rate Transition1/1
  Delay3/1 -> Add/2
  HiR_0/1 -> HwModeRegister/1
  HiR_2/1 -> HwModeRegister2/1
  HiR_4/1 -> HwModeRegister4/1
  PipelineRegister/1 -> Add/1
  PipelineRegister1/1 -> Add1/1
  delayMatch/1 -> Add1/2
  Rate Transition/1 -> Delay1/1, HwModeRegister3/1
  Rate Transition1/1 -> HwModeRegister5/1
  In_HiR_e/1 -> Delay/1, HwModeRegister1/1
  PipelineRegister2/1 -> delayMatch/1
  Multiply/1 -> PipelineRegister/1
  HwModeRegister/1 -> Multiply/1
  HwModeRegister1/1 -> Multiply/2
  Multiply1/1 -> PipelineRegister1/1
  HwModeRegister2/1 -> Multiply1/1
  HwModeRegister3/1 -> Multiply1/2
  Multiply2/1 -> PipelineRegister2/1
  HwModeRegister4/1 -> Multiply2/1
  HwModeRegister5/1 -> Multiply2/2

== system gm_final_heart_sym3_3_Level_fixed/DWT_sym3_3_Level/1st_Level_Recon1/HiR_Odd ==
  In_HiR_o : Inport  OutDataTypeStr=fixdt(1, 16, 28)  PortDimensions=1  SampleTime=2.26757369614512e-05
  Add : Sum  AccumDataTypeStr=fixdt(1, 16, 29)  OutDataTypeStr=fixdt(1, 16, 29)  SampleTime=2.26757369614512e-05
  Add1 : Sum  AccumDataTypeStr=fixdt(1, 16, 29)  OutDataTypeStr=fixdt(1, 16, 29)  SampleTime=2.26757369614512e-05
  Delay : Delay  DelayLength=double(1)  InitialCondition=0  SampleTime=2.26757369614512e-05
  Delay1 : Delay  DelayLength=double(1)  InitialCondition=0  SampleTime=2.26757369614512e-05
  Delay3 : Delay  DelayLength=double(1)  InitialCondition=0  SampleTime=2.26757369614512e-05
  HiR_1 : Constant  Value=0.08544158935546875  OutDataTypeStr=fixdt(0, 16, 19)  SampleTime=2.26757369614512e-05
  HiR_3 : Constant  Value=-0.4598846435546875  OutDataTypeStr=fixdt(1, 16, 16)  SampleTime=2.26757369614512e-05
  HiR_5 : Constant  Value=-0.332672119140625  OutDataTypeStr=fixdt(1, 16, 16)  SampleTime=2.26757369614512e-05
  HwModeRegister{,1..5} (6 alike) : Delay  DelayLength=double(1)  InitialCondition=0  SampleTime=2.26757369614512e-05
  Multiply : Product  Inputs=**  OutDataTypeStr=fixdt(1, 16, 31)  SampleTime=2.26757369614512e-05
  Multiply1 : Product  Inputs=**  OutDataTypeStr=fixdt(1, 16, 29)  SampleTime=2.26757369614512e-05
  Multiply2 : Product  Inputs=**  OutDataTypeStr=fixdt(1, 16, 30)  SampleTime=2.26757369614512e-05
  PipelineRegister : Delay  DelayLength=double(1)  InitialCondition=0  SampleTime=2.26757369614512e-05
  PipelineRegister1 : Delay  DelayLength=double(1)  InitialCondition=0  SampleTime=2.26757369614512e-05
  PipelineRegister2 : Delay  DelayLength=double(1)  InitialCondition=0  SampleTime=2.26757369614512e-05
  Rate Transition : hdlmdlgenlib/Buffer
      settings: SourceProductBaseCode=SL
  Rate Transition1 : hdlmdlgenlib/Buffer
      settings: SourceProductBaseCode=SL
  delayMatch : Delay  DelayLength=double(1)  InitialCondition=0  SampleTime=2.26757369614512e-05
  Out_HiR_o : Outport  OutDataTypeStr=fixdt(1,16,29)  SampleTime=2.26757369614512e-05  VectorParamsAs1DForOutWhenUnconnected=off
  wires:
  Add/1 -> Out_HiR_o/1
  Add1/1 -> Delay3/1
  Delay/1 -> Rate Transition/1
  Delay1/1 -> Rate Transition1/1
  Delay3/1 -> Add/2
  HiR_1/1 -> HwModeRegister/1
  HiR_3/1 -> HwModeRegister2/1
  HiR_5/1 -> HwModeRegister4/1
  PipelineRegister/1 -> Add/1
  PipelineRegister1/1 -> Add1/1
  delayMatch/1 -> Add1/2
  Rate Transition/1 -> Delay1/1, HwModeRegister3/1
  Rate Transition1/1 -> HwModeRegister5/1
  In_HiR_o/1 -> Delay/1, HwModeRegister1/1
  PipelineRegister2/1 -> delayMatch/1
  Multiply/1 -> PipelineRegister/1
  HwModeRegister/1 -> Multiply/1
  HwModeRegister1/1 -> Multiply/2
  Multiply1/1 -> PipelineRegister1/1
  HwModeRegister2/1 -> Multiply1/1
  HwModeRegister3/1 -> Multiply1/2
  Multiply2/1 -> PipelineRegister2/1
  HwModeRegister4/1 -> Multiply2/1
  HwModeRegister5/1 -> Multiply2/2

== system gm_final_heart_sym3_3_Level_fixed/DWT_sym3_3_Level/1st_Level_Recon1/LoR_Even ==
  In_LoR_e : Inport  OutDataTypeStr=fixdt(1, 16, 24)  PortDimensions=1  SampleTime=2.26757369614512e-05
  Add : Sum  AccumDataTypeStr=fixdt(1, 16, 24)  OutDataTypeStr=fixdt(1, 16, 24)  SampleTime=2.26757369614512e-05
  Add1 : Sum  AccumDataTypeStr=fixdt(1, 16, 25)  OutDataTypeStr=fixdt(1, 16, 25)  SampleTime=2.26757369614512e-05
  Delay : Delay  DelayLength=double(1)  InitialCondition=0  SampleTime=2.26757369614512e-05
  Delay1 : Delay  DelayLength=double(1)  InitialCondition=0  SampleTime=2.26757369614512e-05
  Delay3 : Delay  DelayLength=double(1)  InitialCondition=0  SampleTime=2.26757369614512e-05
  HwModeRegister{,1..5} (6 alike) : Delay  DelayLength=double(1)  InitialCondition=0  SampleTime=2.26757369614512e-05
  LoR_0 : Constant  Value=0.332672119140625  OutDataTypeStr=fixdt(0, 16, 17)  SampleTime=2.26757369614512e-05
  LoR_2 : Constant  Value=0.45987701416015625  OutDataTypeStr=fixdt(0, 16, 17)  SampleTime=2.26757369614512e-05
  LoR_4 : Constant  Value=-0.08544158935546875  OutDataTypeStr=fixdt(1, 16, 18)  SampleTime=2.26757369614512e-05
  Multiply : Product  Inputs=**  OutDataTypeStr=fixdt(1, 16, 25)  SampleTime=2.26757369614512e-05
  Multiply1 : Product  Inputs=**  OutDataTypeStr=fixdt(1, 16, 25)  SampleTime=2.26757369614512e-05
  Multiply2 : Product  Inputs=**  OutDataTypeStr=fixdt(1, 16, 27)  SampleTime=2.26757369614512e-05
  PipelineRegister : Delay  DelayLength=double(1)  InitialCondition=0  SampleTime=2.26757369614512e-05
  PipelineRegister1 : Delay  DelayLength=double(1)  InitialCondition=0  SampleTime=2.26757369614512e-05
  PipelineRegister2 : Delay  DelayLength=double(1)  InitialCondition=0  SampleTime=2.26757369614512e-05
  Rate Transition : hdlmdlgenlib/Buffer
      settings: SourceProductBaseCode=SL
  Rate Transition1 : hdlmdlgenlib/Buffer
      settings: SourceProductBaseCode=SL
  delayMatch : Delay  DelayLength=double(1)  InitialCondition=0  SampleTime=2.26757369614512e-05
  Out_LoR_e : Outport  OutDataTypeStr=fixdt(1,16,24)  SampleTime=2.26757369614512e-05  VectorParamsAs1DForOutWhenUnconnected=off
  wires:
  Add/1 -> Out_LoR_e/1
  Add1/1 -> Delay3/1
  Delay/1 -> Rate Transition/1
  Delay1/1 -> Rate Transition1/1
  Delay3/1 -> Add/2
  LoR_0/1 -> HwModeRegister/1
  LoR_2/1 -> HwModeRegister2/1
  LoR_4/1 -> HwModeRegister4/1
  PipelineRegister/1 -> Add/1
  PipelineRegister1/1 -> Add1/1
  delayMatch/1 -> Add1/2
  Rate Transition/1 -> Delay1/1, HwModeRegister3/1
  Rate Transition1/1 -> HwModeRegister5/1
  In_LoR_e/1 -> Delay/1, HwModeRegister1/1
  PipelineRegister2/1 -> delayMatch/1
  Multiply/1 -> PipelineRegister/1
  HwModeRegister/1 -> Multiply/1
  HwModeRegister1/1 -> Multiply/2
  Multiply1/1 -> PipelineRegister1/1
  HwModeRegister2/1 -> Multiply1/1
  HwModeRegister3/1 -> Multiply1/2
  Multiply2/1 -> PipelineRegister2/1
  HwModeRegister4/1 -> Multiply2/1
  HwModeRegister5/1 -> Multiply2/2

== system gm_final_heart_sym3_3_Level_fixed/DWT_sym3_3_Level/1st_Level_Recon1/LoR_Odd ==
  In_LoR_o : Inport  OutDataTypeStr=fixdt(1, 16, 24)  PortDimensions=1  SampleTime=2.26757369614512e-05
  Add : Sum  AccumDataTypeStr=fixdt(1, 16, 24)  OutDataTypeStr=fixdt(1, 16, 24)  SampleTime=2.26757369614512e-05
  Add1 : Sum  AccumDataTypeStr=fixdt(1, 16, 26)  OutDataTypeStr=fixdt(1, 16, 27)  SampleTime=2.26757369614512e-05
  Delay : Delay  DelayLength=double(1)  InitialCondition=0  SampleTime=2.26757369614512e-05
  Delay1 : Delay  DelayLength=double(1)  InitialCondition=0  SampleTime=2.26757369614512e-05
  Delay3 : Delay  DelayLength=double(1)  InitialCondition=0  SampleTime=2.26757369614512e-05
  HwModeRegister{,1..5} (6 alike) : Delay  DelayLength=double(1)  InitialCondition=0  SampleTime=2.26757369614512e-05
  LoR_1 : Constant  Value=0.806884765625  OutDataTypeStr=fixdt(0, 16, 16)  SampleTime=2.26757369614512e-05
  LoR_3 : Constant  Value=-0.135009765625  OutDataTypeStr=fixdt(1, 16, 17)  SampleTime=2.26757369614512e-05
  LoR_5 : Constant  Value=0.03522586822509765625  OutDataTypeStr=fixdt(0, 16, 20)  SampleTime=2.26757369614512e-05
  Multiply : Product  Inputs=**  OutDataTypeStr=fixdt(1, 16, 24)  SampleTime=2.26757369614512e-05
  Multiply1 : Product  Inputs=**  OutDataTypeStr=fixdt(1, 16, 26)  SampleTime=2.26757369614512e-05
  Multiply2 : Product  Inputs=**  OutDataTypeStr=fixdt(1, 16, 28)  SampleTime=2.26757369614512e-05
  PipelineRegister : Delay  DelayLength=double(1)  InitialCondition=0  SampleTime=2.26757369614512e-05
  PipelineRegister1 : Delay  DelayLength=double(1)  InitialCondition=0  SampleTime=2.26757369614512e-05
  PipelineRegister2 : Delay  DelayLength=double(1)  InitialCondition=0  SampleTime=2.26757369614512e-05
  Rate Transition : hdlmdlgenlib/Buffer
      settings: SourceProductBaseCode=SL
  Rate Transition1 : hdlmdlgenlib/Buffer
      settings: SourceProductBaseCode=SL
  delayMatch : Delay  DelayLength=double(1)  InitialCondition=0  SampleTime=2.26757369614512e-05
  Out_LoR_o : Outport  OutDataTypeStr=fixdt(1,16,24)  SampleTime=2.26757369614512e-05  VectorParamsAs1DForOutWhenUnconnected=off
  wires:
  Add/1 -> Out_LoR_o/1
  Add1/1 -> Delay3/1
  Delay/1 -> Rate Transition/1
  Delay1/1 -> Rate Transition1/1
  Delay3/1 -> Add/2
  LoR_1/1 -> HwModeRegister/1
  LoR_3/1 -> HwModeRegister2/1
  LoR_5/1 -> HwModeRegister4/1
  PipelineRegister/1 -> Add/1
  PipelineRegister1/1 -> Add1/1
  delayMatch/1 -> Add1/2
  Rate Transition/1 -> Delay1/1, HwModeRegister3/1
  Rate Transition1/1 -> HwModeRegister5/1
  In_LoR_o/1 -> Delay/1, HwModeRegister1/1
  PipelineRegister2/1 -> delayMatch/1
  Multiply/1 -> PipelineRegister/1
  HwModeRegister/1 -> Multiply/1
  HwModeRegister1/1 -> Multiply/2
  Multiply1/1 -> PipelineRegister1/1
  HwModeRegister2/1 -> Multiply1/1
  HwModeRegister3/1 -> Multiply1/2
  Multiply2/1 -> PipelineRegister2/1
  HwModeRegister4/1 -> Multiply2/1
  HwModeRegister5/1 -> Multiply2/2

== system gm_final_heart_sym3_3_Level_fixed/DWT_sym3_3_Level/1st_Level_Recon2/HiR_Even ==
  In_HiR_e : Inport  OutDataTypeStr=fixdt(1, 16, 28)  PortDimensions=1  SampleTime=2.26757369614512e-05
  Add : Sum  AccumDataTypeStr=fixdt(1, 16, 28)  OutDataTypeStr=fixdt(1, 16, 28)  SampleTime=2.26757369614512e-05
  Add1 : Sum  AccumDataTypeStr=fixdt(1, 16, 28)  OutDataTypeStr=fixdt(1, 16, 28)  SampleTime=2.26757369614512e-05
  Delay : Delay  DelayLength=double(1)  InitialCondition=0  SampleTime=2.26757369614512e-05
  Delay1 : Delay  DelayLength=double(1)  InitialCondition=0  SampleTime=2.26757369614512e-05
  Delay3 : Delay  DelayLength=double(1)  InitialCondition=0  SampleTime=2.26757369614512e-05
  HiR_0 : Constant  Value=0.03522586822509765625  OutDataTypeStr=fixdt(0, 16, 20)  SampleTime=2.26757369614512e-05
  HiR_2 : Constant  Value=-0.135009765625  OutDataTypeStr=fixdt(1, 16, 17)  SampleTime=2.26757369614512e-05
  HiR_4 : Constant  Value=0.806884765625  OutDataTypeStr=fixdt(0, 16, 16)  SampleTime=2.26757369614512e-05
  HwModeRegister{,1..5} (6 alike) : Delay  DelayLength=double(1)  InitialCondition=0  SampleTime=2.26757369614512e-05
  Multiply : Product  Inputs=**  OutDataTypeStr=fixdt(1, 16, 33)  SampleTime=2.26757369614512e-05
  Multiply1 : Product  Inputs=**  OutDataTypeStr=fixdt(1, 16, 31)  SampleTime=2.26757369614512e-05
  Multiply2 : Product  Inputs=**  OutDataTypeStr=fixdt(1, 16, 28)  SampleTime=2.26757369614512e-05
  PipelineRegister : Delay  DelayLength=double(1)  InitialCondition=0  SampleTime=2.26757369614512e-05
  PipelineRegister1 : Delay  DelayLength=double(1)  InitialCondition=0  SampleTime=2.26757369614512e-05
  PipelineRegister2 : Delay  DelayLength=double(1)  InitialCondition=0  SampleTime=2.26757369614512e-05
  Rate Transition : hdlmdlgenlib/Buffer
      settings: SourceProductBaseCode=SL
  Rate Transition1 : hdlmdlgenlib/Buffer
      settings: SourceProductBaseCode=SL
  delayMatch : Delay  DelayLength=double(1)  InitialCondition=0  SampleTime=2.26757369614512e-05
  Out_HiR_e : Outport  OutDataTypeStr=fixdt(1,16,28)  SampleTime=2.26757369614512e-05  VectorParamsAs1DForOutWhenUnconnected=off
  wires:
  Add/1 -> Out_HiR_e/1
  Add1/1 -> Delay3/1
  Delay/1 -> Rate Transition/1
  Delay1/1 -> Rate Transition1/1
  Delay3/1 -> Add/2
  HiR_0/1 -> HwModeRegister/1
  HiR_2/1 -> HwModeRegister2/1
  HiR_4/1 -> HwModeRegister4/1
  PipelineRegister/1 -> Add/1
  PipelineRegister1/1 -> Add1/1
  delayMatch/1 -> Add1/2
  Rate Transition/1 -> Delay1/1, HwModeRegister3/1
  Rate Transition1/1 -> HwModeRegister5/1
  In_HiR_e/1 -> Delay/1, HwModeRegister1/1
  PipelineRegister2/1 -> delayMatch/1
  Multiply/1 -> PipelineRegister/1
  HwModeRegister/1 -> Multiply/1
  HwModeRegister1/1 -> Multiply/2
  Multiply1/1 -> PipelineRegister1/1
  HwModeRegister2/1 -> Multiply1/1
  HwModeRegister3/1 -> Multiply1/2
  Multiply2/1 -> PipelineRegister2/1
  HwModeRegister4/1 -> Multiply2/1
  HwModeRegister5/1 -> Multiply2/2
